simulink model "IfElseLogic"  (R2013a)
settings: Solver=ode45  StartTime=0.0  StopTime=10.0  RelTol=1e-3
settings Model: Creator=ajdin  LastModifiedBy=ajdin

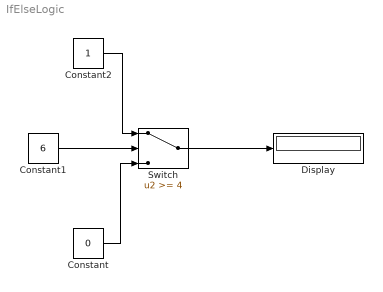
== system IfElseLogic ==
  Constant : Constant  Value=0
  Constant1 : Constant  Value=6
  Constant2 : Constant
  Display : Display
  Switch : Switch  Threshold=4
  wires:
  Switch/1 -> Display/1
  Constant1/1 -> Switch/2
  Constant/1 -> Switch/3
  Constant2/1 -> Switch/1
